simulink model "sim_passive_hc_ssrf_verify"  (R2020b)
settings: Solver=VariableStepAuto  StartTime=0.0  StopTime=10.0  RelTol=1e-3
InitFcn:
  | %————————————————————————————
  | %自变量
  | %————————————————————————————
  | IB = 300/1000;
  | fF = -0/180*pi;
  | X = 0;
  | delf = 22e3;
  | thetaL = 0/180*pi;
  | wa = 2*pi*1e3;
  | wp = 2*pi*1e3;
  | KCa = 0;
  | KCp = 0;
  | %————————————————————————————
  | %常量（不同模式不同）
  | %————————————————————————————
  | VA = 5.4e6;
  | %Vp = 1.8e6;
  | %————————————————————————————
  | %常量
  | %————————————————————————————
  | RLp_ratio_Qp = 87.5;
  | Qp = 1e10;
  | RLp = Qp*RLp_ratio_Qp*2;
  | R0_ratio_Q0 = 89;
  | Q0 = 1.2e9;
  | QL = 1.6e5;
  | R0 = 2.136e11;
  | RL = 2.848e7;
  | frf = 500e6;
  | n = 3;
  | fhrf = frf*n;
  | U_ratio_e =1.44e6;
  | sigma = 2*pi*frf/(2*QL);
  | sigmap = 2*pi*fhrf/(2*Qp);
  | DRFB_delay = 0;
  | mc_delay = 0;
  | %————————————————————————————
  | %计算得出以下物理量
  | %————————————————————————————
  | Gf = X/RL;
  | I0 = VA/RL;
  | Y = IB/I0;
  | VP = IB*RLp_ratio_Qp*fhrf/delf;
  | fLp = acos(VP/RLp/IB);
  | fs = acos((U_ratio_e+VP*cos(fLp))/(VA));
  | %fL = atan(IB*tan(thetaL)*cos(fs)/I0+tan(thetaL)-IB*sin(fs)/I0);
  | %FL = atan(tan(fL)+X*(sin(fF)-cos(fF)*tan(fL)));
  | fL = -atan(Y*sin(fs)-X*sin(fF)-(1+Y*cos(fs)-X*cos(fF))*tan(thetaL));
  | thetaT = -atan((VA*cos(fs)-VP*cos(fLp))/(VA*sin(fs)-VP*sin(fLp)));
  | VT = sqrt(VA^2+VP^2-2*VA*VP*cos(fs-fLp));
  | T0 = 432/3/1e8;
  | ws = sqrt(2*pi*(4.2227e-4)*720*VT*cos(-thetaT)/T0/T0/3.5/1e9);
  | alpha = U_ratio_e/T0/3.5/1e9;
  | %————————————————————————————
  | %传递函数各分子分母
  | %————————————————————————————
  | syms s
  | %sdelay = 1-s*DRFB_delay+s^2*DRFB_delay^2/2-s^3*DRFB_delay^3/6+s^4*DRFB_delay^4/24;
  | sdelay_DRFB = 1-s*DRFB_delay;
  | sdelay_mc = 1-s*mc_delay;
  | G_fenmu = s^2+2*sigma*s+sigma^2*(sec(fL))^2;
  | Gaa_fenzi = sigma*s+sigma^2*(1+(tan(fL))^2);
  | Gpp_fenzi = Gaa_fenzi;
  | Gpa_fenzi = sigma*tan(fL)*s;
  | Gap_fenzi = -Gpa_fenzi;
  | Gaa = Gaa_fenzi/G_fenmu;
  | Gpp = Gpp_fenzi/G_fenmu;
  | Gpa = Gpa_fenzi/G_fenmu;
  | Gap = Gap_fenzi/G_fenmu;
  | IT = I0/cos(fL);
  | IG = I0*(1-X*cos(fF)+Y*cos(fs))/cos(thetaL);
  | GppB = IB/IT*(-Gap*sin(fs-fL)-Gpp*cos(fs-fL));
  | GpaB = IB/IT*(-Gaa*sin(fs-fL)-Gpa*cos(fs-fL));
  | GppG = IG/IT*(Gap*sin(thetaL-fL)+Gpp*cos(thetaL-fL));
  | GpaG = IG/IT*(Gaa*sin(thetaL-fL)+Gpa*cos(thetaL-fL));
  | GaaG = GppG;GapG = -GpaG;
  | GppF = sdelay_DRFB*X*IB/IT*(Gap*sin(fF-fL)+Gpp*cos(fF-fL));
  | GpaF = sdelay_DRFB*X*IB/IT*(Gaa*sin(fF-fL)+Gpa*cos(fF-fL));
  | GaaF = GppF;GapF = -GpaF;
  | [GppB_fenzi,GppB_fenmu] = numden(GppB);[GpaB_fenzi,GpaB_fenmu] = numden(GpaB);
  | [GppG_fenzi,GppG_fenmu] = numden(GppG);[GpaG_fenzi,GpaG_fenmu] = numden(GpaG);
  | [GaaG_fenzi,GaaG_fenmu] = numden(GaaG);[GapG_fenzi,GapG_fenmu] = numden(GapG);
  | [GppF_fenzi,GppF_fenmu] = numden(GppF);[GpaF_fenzi,GpaF_fenmu] = numden(GpaF);
  | [GaaF_fenzi,GaaF_fenmu] = numden(GaaF);[GapF_fenzi,GapF_fenmu] = numden(GapF);
  | GppB_fz = sym2poly(GppB_fenzi);GppB_fm = sym2poly(GppB_fenmu);
  | GpaB_fz = sym2poly(GpaB_fenzi);GpaB_fm = sym2poly(GpaB_fenmu);
  | GppG_fz = sym2poly(GppG_fenzi);GppG_fm = sym2poly(GppG_fenmu);
  | GpaG_fz = sym2poly(GpaG_fenzi);GpaG_fm = sym2poly(GpaG_fenmu);
  | GaaG_fz = sym2poly(GaaG_fenzi);GaaG_fm = sym2poly(GaaG_fenmu);
  | GapG_fz = sym2poly(GapG_fenzi);GapG_fm = sym2poly(GapG_fenmu);
  | GppF_fz = sym2poly(GppF_fenzi);GppF_fm = sym2poly(GppF_fenmu);
  | GpaF_fz = sym2poly(GpaF_fenzi);GpaF_fm = sym2poly(GpaF_fenmu);
  | GaaF_fz = sym2poly(GaaF_fenzi);GaaF_fm = sym2poly(GaaF_fenmu);
  | GapF_fz = sym2poly(GapF_fenzi);GapF_fm = sym2poly(GapF_fenmu);
  | 
  | 
  | h_fm = [1 2*sigmap sigmap^2*(1+(tan(fLp))^2)];
  | B_fm = [1 alpha ws^2];
  | GpaBP_fz = [sigmap*tan(fLp) 0];
  | GppBP_fz = [sigmap sigmap^2*(1+(tan(fLp))^2)];
  | %Cp_fz = wp;Cp_fm = [1 wp];
  | %Ca_fz = wa;Ca_fm = [1 wa];
  | Cp_fz = [-mc_delay*wp wp];Cp_fm = [1 wp];
  | Ca_fz = [-mc_delay*wa wa];Ca_fm = [1 wa];
  | %————————————————————————————
  | %传递函数计算
  | %————————————————————————————
  | B = tf(ws^2,B_fm);
  | GpaB = tf(GpaB_fz,GpaB_fm);GppB = tf(GppB_fz,GppB_fm);
  | GpaG = tf(GpaG_fz,GpaG_fm);GppG = tf(GppG_fz,GppG_fm);
  | GpaF = tf(GpaF_fz,GpaF_fm);GppF = tf(GppF_fz,GppF_fm);
  | GapG = -GpaG;GaaG = GppG;
  | GapF = -GpaF;GaaF = GppF;
  | GpaBP = tf(GpaBP_fz,h_fm);GppBP = tf(GppBP_fz,h_fm);
  | Gab = (-cos(thetaT-fs)-sin(thetaT-fs)*tan(thetaT))*VA/VT;
  | Gpb = (-sin(thetaT-fs)+cos(thetaT-fs)*tan(thetaT))*VA/VT;
  | GabP = (cos(thetaT-fLp)+sin(thetaT-fLp)*tan(thetaT))*VP/VT;
  | GpbP = (sin(thetaT-fLp)-cos(thetaT-fLp)*tan(thetaT))*VP/VT;
settings Model: Creator=Administrator  LastModifiedBy=Administrator

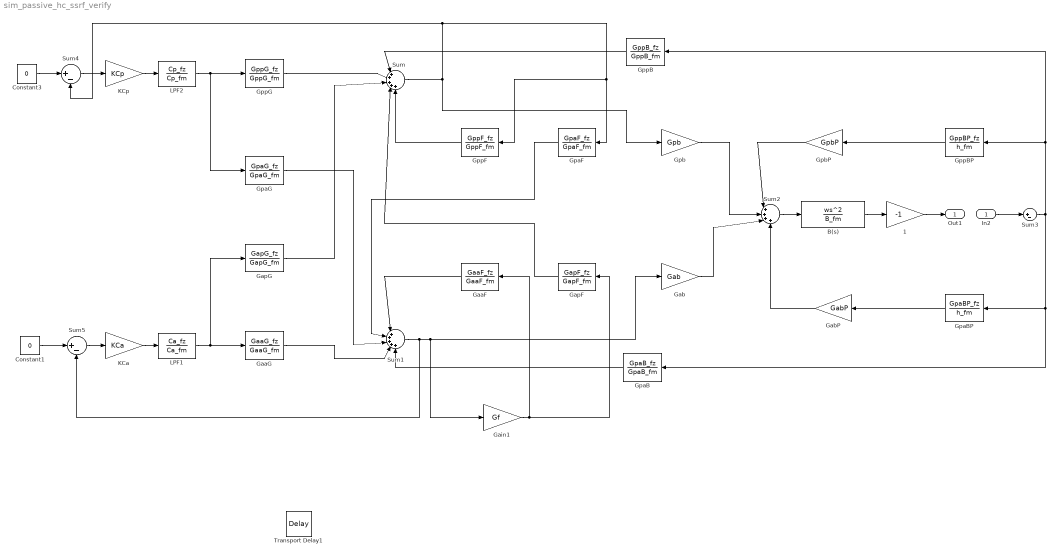
== system sim_passive_hc_ssrf_verify ==
  In2 : Inport
  "  1" : Gain  Gain=-1
  B(s) : TransferFcn  Numerator=ws^2  Denominator=B_fm
  Constant1 : Constant  Value=0
  Constant3 : Constant  Value=0
  GaaF : TransferFcn  Numerator=GaaF_fz  Denominator=GaaF_fm
  GaaG : TransferFcn  Numerator=GaaG_fz  Denominator=GaaG_fm
  Gab : Gain  Gain=Gab
  GabP : Gain  Gain=GabP
  Gain1 : Gain  Gain=Gf
  GapF : TransferFcn  Numerator=GapF_fz  Denominator=GapF_fm
  GapG : TransferFcn  Numerator=GapG_fz  Denominator=GapG_fm
  GpaB : TransferFcn  Numerator=GpaB_fz  Denominator=GpaB_fm
  GpaBP : TransferFcn  Numerator=GpaBP_fz  Denominator=h_fm
  GpaF : TransferFcn  Numerator=GpaF_fz  Denominator=GpaF_fm
  GpaG : TransferFcn  Numerator=GpaG_fz  Denominator=GpaG_fm
  Gpb : Gain  Gain=Gpb
  GpbP : Gain  Gain=GpbP
  GppB : TransferFcn  Numerator=GppB_fz  Denominator=GppB_fm
  GppBP : TransferFcn  Numerator=GppBP_fz  Denominator=h_fm
  GppF : TransferFcn  Numerator=GppF_fz  Denominator=GppF_fm
  GppG : TransferFcn  Numerator=GppG_fz  Denominator=GppG_fm
  KCa : Gain  Gain=KCa
  KCp : Gain  Gain=KCp
  LPF1 : TransferFcn  Numerator=Ca_fz  Denominator=Ca_fm
  LPF2 : TransferFcn  Numerator=Cp_fz  Denominator=Cp_fm
  Sum : Sum  Inputs=|+++++
  Sum1 : Sum  Inputs=|+++++
  Sum2 : Sum  Inputs=|++++
  Sum3 : Sum  Inputs=|+-
  Sum4 : Sum  Inputs=|+-
  Sum5 : Sum  Inputs=|+-
  Transport Delay1 : TransportDelay  DelayTime=DRFB_delay  PadeOrder=1
  Out1 : Outport
  wires:
  GppB/1 -> Sum/1
  GpaB/1 -> Sum1/5
  GpaG/1 -> Sum1/3
  GapG/1 -> Sum/3
  Sum2/1 -> B(s)/1
  GaaF/1 -> Sum1/1
  Constant1/1 -> Sum5/1
  GapF/1 -> Sum/4
  KCp/1 -> LPF2/1
  KCa/1 -> LPF1/1
  Sum4/1 -> KCp/1
  GabP/1 -> Sum2/4
  Gain1/1 -> GaaF/1, GapF/1
  Gab/1 -> Sum2/3
  GppG/1 -> Sum/2
  Constant3/1 -> Sum4/1
  GaaG/1 -> Sum1/4
  Sum3/1 -> GpaB/1, GpaBP/1, GppB/1, GppBP/1
  GppF/1 -> Sum/5
  Sum5/1 -> KCa/1
  GpaF/1 -> Sum1/2
  In2/1 -> Sum3/1
  GpbP/1 -> Sum2/1
  LPF2/1 -> GpaG/1, GppG/1
  GpaBP/1 -> GabP/1
  LPF1/1 -> GaaG/1, GapG/1
  Gpb/1 -> Sum2/2
  GppBP/1 -> GpbP/1
  Sum/1 -> Sum4/2, GppF/1, GpaF/1, Gpb/1
  Sum1/1 -> Sum5/2, Gain1/1, Gab/1
  B(s)/1 -> "  1"/1
  "  1"/1 -> Out1/1
